simulink model "turbine"  (R2024a)
settings: Solver=VariableStepAuto  StartTime=0.0  StopTime=30  RelTol=1e-3
undefined symbols (not defined in the file): joinTheResistance
libraries: spsDCMachineLib x1, spsCurrentMeasurementLib x1, spsSeriesRLCBranchLib x1, spsVoltageMeasurementLib x1, spsWindTurbineLib x1, sps_lib x1
settings Model: Creator=emanuele  LastModifiedBy=emanuele

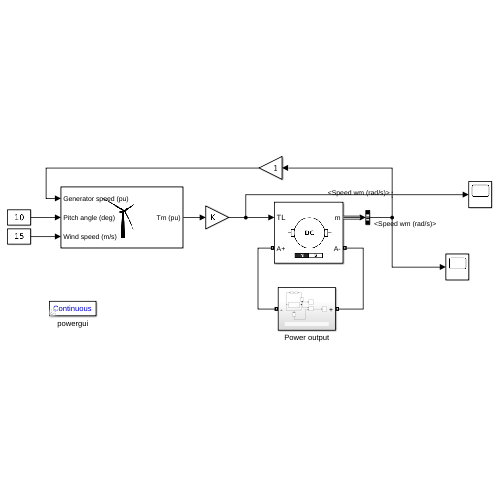
[thumbnail: Simulink's stored preview of the top-level diagram]
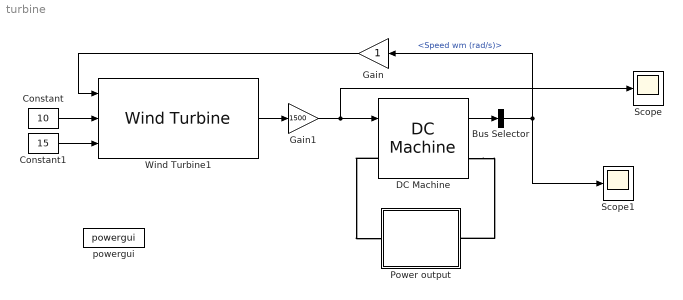
== system turbine ==
  Bus Selector : BusSelector  OutputSignals=Speed wm (rad/s)
  Constant : Constant  Value=10
  Constant1 : Constant  Value=15
  DC Machine : spsDCMachineLib/DC Machine  PresetModel=No  MechanicalLoad=Torque TL  FieldType=Permanent magnet  ShowDetailedParameters=on  MeasurementBus=off  RLa="[ 0.6  0.012]"  RLf="[ 240  120]"  Laf=1.8  MachineConstant=Torque constant (N.m/A)  Ke=1.8  Kt=1.8  J=1  Bm=0  Tf=0  w0=1  Ifinit=1  TsPowergui=0  TsBlock=-1
  Gain : Gain
  Gain1 : Gain  Gain=1500
  Power output : Subsystem
  Scope : Scope
  Scope1 : Scope
  Wind Turbine1 : spsWindTurbineLib/Wind Turbine  Pnom=1500  Pelec_base=1500/0.9  wind_base=12  P_wind_base=0.8  speed_nom=1.2  pitch_angle=0  c1_c6="[0.51763          116          0.4            5           21     0.006795]"  cp_nom=0.48  lambda_nom=8.1
  powergui : sps_lib/powergui  Priority=1  SimulationMode=Continuous  SampleTime=50e-6  frequency=60  Iterations=50  frequencyindice=0  Pbase=100e6  ErrMax=1e-4  UnitsV=kV  UnitsW=MW  buscounter=0  FunctionMessages=off  echomessages=off  EnableUseOfTLC=off  CurrentSourceSwitches=off  DisableSnubberDevices=off  DisableRonSwitches=off  DisableVfSwitches=off  DisplayEquations=off  AutomaticDiscreteSolvers=off  SolverType=Tustin/Backward Euler (TBE)  Interpol=off  ExternalGateDelay=off  methode=off  Ts=100  x0status=blocks  SPID=on  SwTol=0  HookPort=off  NonlinearTolerance=1e-4  nMaxIteration=100  ContinueOnMaxIteration=off  RestoreLinks=warning  ResistiveCurrentMeasurement=off  Frange=[0:2:500]  Ylog=off  Xlog=on  ShowGrid=off  save=off  variable=ZData  structure=0  ZoomFFT=off  StartTime=0.0  cycles=1  DisplayStyle=1  fundamental=60  FreqAxis=off  MaxFrequency=1000  frequencyindicesteady=1  RmsSteady=1  display=off
  wires:
  Constant/1 -> Wind Turbine1/2
  Constant1/1 -> Wind Turbine1/3
  Wind Turbine1/1 -> Gain1/1
  DC Machine/1 -> Bus Selector/1
  Bus Selector/1 -> Gain/1, Scope1/1  "<Speed wm (rad/s)>"
  Gain/1 -> Wind Turbine1/1
  Gain1/1 -> DC Machine/1, Scope/1
  connections:
  DC Machine/LConn1 -- Power output/RConn1
  DC Machine/RConn1 -- Power output/LConn1

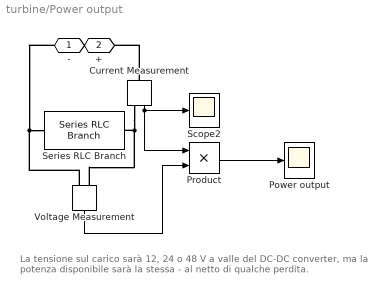
== system turbine/Power output ==
  note: La tensione sul carico sarà 12, 24 o 48 V a valle del DC-DC converter,
      | ma la potenza disponibile sarà la stessa - al netto di qualche perdita.
  Current Measurement : spsCurrentMeasurementLib/Current Measurement  PhasorSimulation=off  OutputType=Complex  PSBequivalent=0
  Power output : Scope
  Product : Product
  Scope2 : Scope
  Series RLC Branch : spsSeriesRLCBranchLib/Series RLC Branch  LConnTagsString=__new0  RConnTagsString=__new0  BranchType=R  Resistance=joinTheResistance  Inductance=0  SetiL0=off  InitialCurrent=0  Capacitance=0  Setx0=off  InitialVoltage=0  Measurements=Branch voltage and current
  Voltage Measurement : spsVoltageMeasurementLib/Voltage Measurement  PhasorSimulation=off  OutputType=Complex  PSBequivalent=0
  - : PMIOPort  Side=Right
  + : PMIOPort  Port=2  Side=Left
  wires:
  Current Measurement/1 -> Scope2/1, Product/1
  Voltage Measurement/1 -> Product/2
  Product/1 -> Power output/1
  connections:
  Voltage Measurement/LConn2 -- -/RConn1 -- Series RLC Branch/LConn1
  Current Measurement/RConn1 -- Voltage Measurement/LConn1 -- Series RLC Branch/RConn1
  Current Measurement/LConn1 -- +/RConn1
